simulink model "RaketeUnterSchwerelosigkeit"  (Simulink 7.1)
settings: Solver=ode45  StartTime=0.0  StopTime=100.0  RelTol=1e-3
settings Model: Creator=Meisel  LastModifiedBy=Meisel

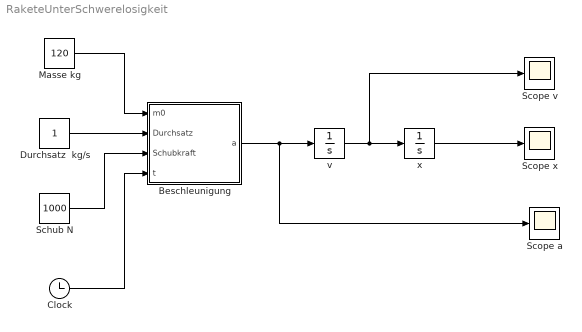
== system RaketeUnterSchwerelosigkeit ==
  Beschleunigung : Stateflow chart
  Clock : Clock
      settings: Decimation=10
  Durchsatz  kg/s : Constant  OutDataType=sfix(16)  OutScaling=2^0
  Masse kg : Constant  Value=120  OutDataType=sfix(16)  OutScaling=2^0
  Schub N : Constant  Value=1000  OutDataType=sfix(16)  OutScaling=2^0
  Scope a : Scope
      settings: TimeRange=100  SaveName=ScopeData2
  Scope v : Scope
  Scope x : Scope
      settings: TimeRange=100
  v : Integrator
  x : Integrator
  wires:
  v/1 -> x/1, Scope v/1
  x/1 -> Scope x/1
  Beschleunigung/1(a) -> v/1, Scope a/1
  Masse kg/1 -> Beschleunigung/1(m0)
  Durchsatz  kg/s/1 -> Beschleunigung/2(Durchsatz)
  Clock/1 -> Beschleunigung/4(t)
  Schub N/1 -> Beschleunigung/3(Schubkraft)

== matlab function Beschleunigung ==
  data: m0 input double; a output double; Durchsatz input double; Schubkraft input double; t input double
function a = fcn(m0, Durchsatz, Schubkraft, t)
% This block supports the Embedded MATLAB subset.
% See the help menu for details. 

a = Schubkraft/(m0-Durchsatz*t);
